simulink model "emodel"  (R2020b)
settings: Solver=VariableStepAuto  StartTime=0.0  StopTime=100  RelTol=1e-3
settings Model: Creator=zceexdu  LastModifiedBy=zceexdu

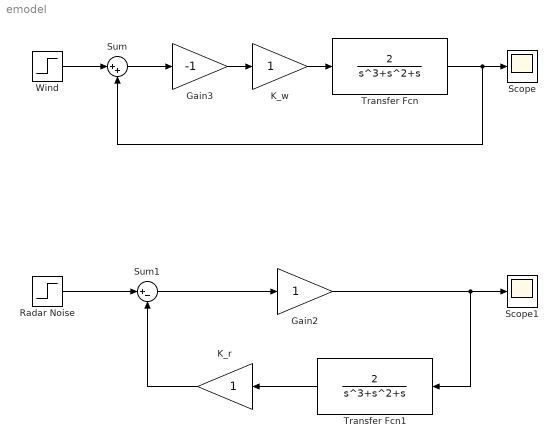
== system emodel ==
  Gain2 : Gain
  Gain3 : Gain  Gain=-1
  K_r : Gain
  K_w : Gain
  Radar Noise : Step
  Scope : Scope
  Scope1 : Scope
  Sum : Sum  Inputs=|++
  Sum1 : Sum  Inputs=|+-
  Transfer Fcn : TransferFcn  Numerator=[2]  Denominator=[1 1 1 0]
  Transfer Fcn1 : TransferFcn  Numerator=[2]  Denominator=[1 1 1 0]
  Wind : Step  SampleTime=0
  wires:
  Wind/1 -> Sum/1
  K_w/1 -> Transfer Fcn/1
  Sum1/1 -> Gain2/1
  Radar Noise/1 -> Sum1/1
  Gain2/1 -> Transfer Fcn1/1, Scope1/1
  Transfer Fcn/1 -> Sum/2, Scope/1
  Transfer Fcn1/1 -> K_r/1
  K_r/1 -> Sum1/2
  Sum/1 -> Gain3/1
  Gain3/1 -> K_w/1
